simulink model "L400_sdofplant"  (R2024b)
settings: Solver=FixedStepAuto  StartTime=0  StopTime=200  FixedStep=5/1000  RelTol=1e-3
model workspace (MAT data in the model file):
  Sig : Simulink.Signal (value not decoded)
  Sig1 : Simulink.Signal (value not decoded)
  Sig2 : Simulink.Signal (value not decoded)
  Sig3 : Simulink.Signal (value not decoded)
  Sig4 : Simulink.Signal (value not decoded)
  Sig5 : Simulink.Signal (value not decoded)
  Sig6 : Simulink.Signal (value not decoded)
undefined symbols (not defined in the file or in its folder): convertTo, datetime, db, Earth, F, Light, MIL, motor, WGS84, WMM2020
libraries: aerolibconvert2 x6, aerolibasang x5, aerolibwind2 x3, aerolibactuator x2, aerolibtransform2 x2, shared6dof x1, matrix_library x1, aerolibatmos2 x1, aerolibgravity2 x1
(part 2 of 3)

== system L400_sdofplant/actuator/aerodynamic/actuator ==
  BusElementIn1 : Inport  PortName=command  Element=DAL
  BusElementIn : Inport  PortName=command  Element=DAL
  BusElementIn2 : Inport  PortName=command  Element=DER
  BusElementIn3 : Inport  PortName=command  Element=DR
  BusElementIn4 : Inport  PortName=command  Element=DEM
  BusElementIn5 : Inport  PortName=command  Element=DEL
  BusElementIn6 : Inport  PortName=command  Element=DFLO
  BusElementIn7 : Inport  PortName=command  Element=DFLI
  BusElementIn8 : Inport  PortName=command  Element=DFRI
  BusElementIn9 : Inport  PortName=command  Element=DFRO
  Data Type Conversion : DataTypeConversion  SaturateOnIntegerOverflow=off  RndMeth=Floor
  Demux : Demux  Outputs=10
  Mux : Mux  Inputs=10
  Saturation : Saturate  UpperLimit=[30,30,30,30,15,15,17,17,17,23]  LowerLimit=[0,0,0,0,-23,-23,-23,-23,-23,-23]
  Signal Specification4 : SignalSpecification  Unit=deg
  Variant Subsystem : Subsystem  Variant=on
  Bus Element Out : Outport  PortName=surface  Element=DFLO
  Bus Element Out1 : Outport  PortName=surface  Element=DFLI
  Bus Element Out2 : Outport  PortName=surface  Element=DFRI
  Bus Element Out3 : Outport  PortName=surface  Element=DFRO
  Bus Element Out4 : Outport  PortName=surface  Element=DAL
  Bus Element Out5 : Outport  PortName=surface  Element=DAR
  Bus Element Out6 : Outport  PortName=surface  Element=DEL
  Bus Element Out7 : Outport  PortName=surface  Element=DEM
  Bus Element Out8 : Outport  PortName=surface  Element=DER
  Bus Element Out9 : Outport  PortName=surface  Element=DR
  wires:
  Mux/1 -> Data Type Conversion/1
  Saturation/1 -> Signal Specification4/1
  Variant Subsystem/1(Out1) -> Demux/1
  Demux/1 -> Bus Element Out/1
  Demux/2 -> Bus Element Out1/1
  Demux/4 -> Bus Element Out3/1
  Demux/3 -> Bus Element Out2/1
  Signal Specification4/1 -> Variant Subsystem/1(In1)
  BusElementIn6/1 -> Mux/1
  BusElementIn7/1 -> Mux/2
  BusElementIn8/1 -> Mux/3
  BusElementIn9/1 -> Mux/4
  BusElementIn3/1 -> Mux/10
  BusElementIn2/1 -> Mux/9
  BusElementIn5/1 -> Mux/7
  BusElementIn4/1 -> Mux/8
  BusElementIn/1 -> Mux/6
  BusElementIn1/1 -> Mux/5
  Demux/5 -> Bus Element Out4/1
  Demux/6 -> Bus Element Out5/1
  Demux/7 -> Bus Element Out6/1
  Demux/8 -> Bus Element Out7/1
  Demux/9 -> Bus Element Out8/1
  Demux/10 -> Bus Element Out9/1
  Data Type Conversion/1 -> Saturation/1

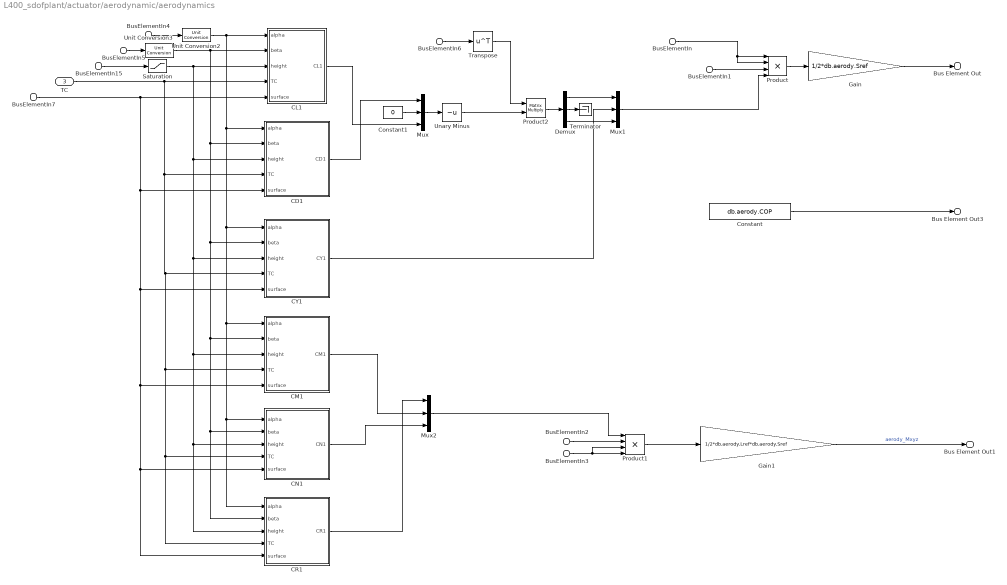
== system L400_sdofplant/actuator/aerodynamic/aerodynamics ==
  BusElementIn7 : Inport  PortName=surface
  BusElementIn : Inport  Port=2  PortName=state  Element=aircraft.airdata.airspeed
  BusElementIn3 : Inport  Port=2  PortName=state  Element=aircraft.airdata.airspeed
  BusElementIn4 : Inport  Port=2  PortName=state  Element=aircraft.airdata.alpha
  BusElementIn5 : Inport  Port=2  PortName=state  Element=aircraft.airdata.beta
  BusElementIn6 : Inport  Port=2  PortName=state  Element=aircraft.airdata.Rwb
  BusElementIn15 : Inport  Port=2  PortName=state  Element=aircraft.position.agl
  BusElementIn1 : Inport  Port=2  PortName=state  Element=environ.atmosphere.density
  BusElementIn2 : Inport  Port=2  PortName=state  Element=environ.atmosphere.density
  TC : Inport  Port=3
  CD1 : Subsystem
  CL1 : Subsystem
  CM1 : Subsystem
  CN1 : Subsystem
  CR1 : Subsystem
  CY1 : Subsystem
  Constant : Constant  Value=db.aerody.COP
  Constant1 : Constant  Value=0
  Demux : Demux  Outputs=3
  Gain : Gain  Gain=1/2*db.aerody.Sref
  Gain1 : Gain  Gain=1/2*db.aerody.Lref*db.aerody.Sref
  Mux : Mux  Inputs=3
  Mux1 : Mux  Inputs=3
  Mux2 : Mux  Inputs=3
  Product : Product  Inputs=4
  Product1 : Product  Inputs=4
  Product2 : Product  Multiplication=Matrix(*)
  Saturation : Saturate  UpperLimit=5.8  LowerLimit=0
  Terminator : Terminator
  Transpose : Math  Operator=transpose
  Unary Minus : UnaryMinus
  Unit Conversion2 : UnitConversion
  Unit Conversion3 : UnitConversion
  Bus Element Out : Outport  PortName=aerody  Element=Fxyz
  Bus Element Out1 : Outport  PortName=aerody  Element=Mxyz
  Bus Element Out3 : Outport  PortName=aerody  Element=Pxyz
  wires:
  BusElementIn/1 -> Product/2, Product/1
  BusElementIn2/1 -> Product1/2
  Constant/1 -> Bus Element Out3/1
  Product1/1 -> Gain1/1
  Product/1 -> Gain/1
  BusElementIn3/1 -> Product1/4, Product1/3
  Mux2/1 -> Product1/1
  BusElementIn1/1 -> Product/3
  Gain1/1 -> Bus Element Out1/1  "aerody_Mxyz"
  Unit Conversion2/1 -> CR1/1(alpha), CN1/1(alpha), CM1/1(alpha), CY1/1(alpha), CD1/1(alpha), CL1/1(alpha)
  BusElementIn7/1 -> CL1/5(surface), CD1/5(surface), CM1/5(surface), CN1/5(surface), CR1/5(surface), CY1/5(surface)
  BusElementIn4/1 -> Unit Conversion2/1
  BusElementIn5/1 -> Unit Conversion3/1
  BusElementIn15/1 -> Saturation/1
  TC/1 -> CM1/4(TC), CN1/4(TC), CR1/4(TC), CY1/4(TC), CD1/4(TC), CL1/4(TC)
  Unit Conversion3/1 -> CM1/2(beta), CN1/2(beta), CR1/2(beta), CY1/2(beta), CD1/2(beta), CL1/2(beta)
  CD1/1(CD1) -> Mux/1
  CL1/1(CL1) -> Mux/3
  Constant1/1 -> Mux/2
  Mux/1 -> Unary Minus/1
  BusElementIn6/1 -> Transpose/1
  Transpose/1 -> Product2/1
  CY1/1(CY1) -> Mux1/2
  Product2/1 -> Demux/1
  Demux/1 -> Mux1/1
  Demux/3 -> Mux1/3
  Demux/2 -> Terminator/1
  Mux1/1 -> Product/4
  CM1/1(CM1) -> Mux2/2
  CR1/1(CR1) -> Mux2/1
  CN1/1(CN1) -> Mux2/3
  Saturation/1 -> CM1/3(height), CN1/3(height), CR1/3(height), CY1/3(height), CD1/3(height), CL1/3(height)
  Unary Minus/1 -> Product2/2
  Gain/1 -> Bus Element Out/1

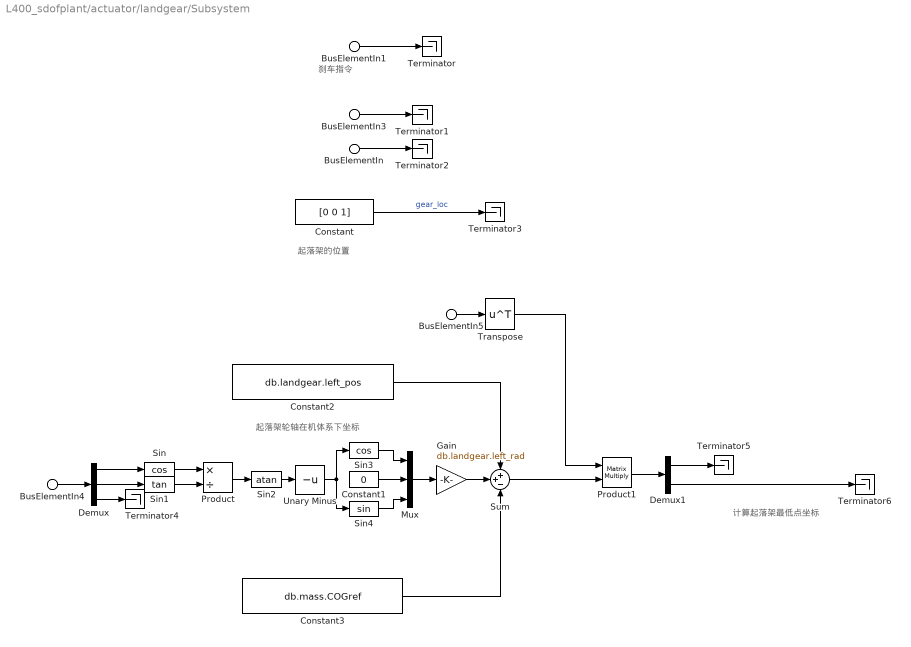
== system L400_sdofplant/actuator/landgear/Subsystem ==
  note: 起落架轮轴在机体系下坐标
  note: 计算起落架最低点坐标
  note: 刹车指令
  note: 起落架的位置
  BusElementIn1 : Inport  PortName=cmd  Element=DB
  BusElementIn : Inport  Port=2  PortName=state  Element=aircraft.position.agl
  BusElementIn3 : Inport  Port=2  PortName=state  Element=aircraft.position.alt
  BusElementIn4 : Inport  Port=2  PortName=state  Element=aircraft.attitude.phi_theta_psi
  BusElementIn5 : Inport  Port=2  PortName=state  Element=aircraft.attitude.Rbe
  Constant : Constant  Value=[0 0 1]
  Constant1 : Constant  Value=0
  Constant2 : Constant  Value=db.landgear.left_pos
  Constant3 : Constant  Value=db.mass.COGref
  Demux : Demux  Outputs=3
  Demux1 : Demux  Outputs=[2, 1]
  Gain : Gain  Gain=db.landgear.left_rad
  Mux : Mux  Inputs=3
  Product : Product  Inputs=*/
  Product1 : Product  Multiplication=Matrix(*)
  Sin : Trigonometry  Operator=cos
  Sin1 : Trigonometry  Operator=tan
  Sin2 : Trigonometry  Operator=atan
  Sin3 : Trigonometry  Operator=cos
  Sin4 : Trigonometry
  Sum : Sum  Inputs=++-
  Terminator{,1..6} (7 alike) : Terminator
  Transpose : Math  Operator=transpose
  Unary Minus : UnaryMinus
  wires:
  Constant/1 -> Terminator3/1  "gear_loc"
  BusElementIn1/1 -> Terminator/1
  BusElementIn3/1 -> Terminator1/1
  BusElementIn/1 -> Terminator2/1
  BusElementIn4/1 -> Demux/1
  Demux/2 -> Sin1/1
  Demux/1 -> Sin/1
  Sin/1 -> Product/1
  Sin1/1 -> Product/2
  Product/1 -> Sin2/1
  Demux/3 -> Terminator4/1
  Sin2/1 -> Unary Minus/1
  Constant1/1 -> Mux/2
  Sin3/1 -> Mux/1
  Sin4/1 -> Mux/3
  Mux/1 -> Gain/1
  BusElementIn5/1 -> Transpose/1
  Transpose/1 -> Product1/1
  Sum/1 -> Product1/2
  Unary Minus/1 -> Sin4/1, Sin3/1
  Constant2/1 -> Sum/1
  Gain/1 -> Sum/2
  Constant3/1 -> Sum/3
  Product1/1 -> Demux1/1
  Demux1/1 -> Terminator5/1
  Demux1/2 -> Terminator6/1

== system L400_sdofplant/force/Subsystem1/For Each Subsystem ==
  Fxyz : Inport  Partition=on  PartitionDimension=2  PartitionWidth=1  PartitionOffset=0
  Mxyz : Inport  Port=2  Partition=on  PartitionDimension=2  PartitionWidth=1  PartitionOffset=0
  Pxyz : Inport  Port=3  Partition=on  PartitionDimension=2  PartitionWidth=1  PartitionOffset=0
  COG : Inport  Port=4
  Cross Product : matrix_library/Cross Product
  For Each : ForEach  DisableCoverage=on
  Sum : Sum  Inputs=|+-
  Sum1 : Sum  Inputs=|++
  M : Outport  ConcatenationDimension=2
  wires:
  Mxyz/1 -> Sum1/2
  Sum/1 -> Cross Product/1
  Fxyz/1 -> Cross Product/2
  Sum1/1 -> M/1
  Cross Product/1 -> Sum1/1
  Pxyz/1 -> Sum/1
  COG/1 -> Sum/2

== system L400_sdofplant/sensor/gps/posix time ==
  Clock : Clock
  Constant : Constant  Value=convertTo(datetime('now','TimeZone','UTC'),'posixtime')
  Gain : Gain  Gain=1e6  OutDataTypeStr=uint64
  Sum : Sum  Inputs=|++
  utc : Outport  Unit=µs
  wires:
  Clock/1 -> Sum/1
  Sum/1 -> Gain/1
  Constant/1 -> Sum/2
  Gain/1 -> utc/1

== system L400_sdofplant/state/Variant Subsystem/Subsystem ==
  h(m) : Inport
  μ(deg) : Inport  Port=2
  l(deg) : Inport  Port=3
  Constant : Constant  Value=[1 0 0]
  Constant1 : Constant  Value=0
  Terminator : Terminator
  Terminator1 : Terminator
  Terminator2 : Terminator
  XYZ(nT) : Outport
  H(nT) : Outport  Port=2
  D(deg) : Outport  Port=3
  I(deg) : Outport  Port=4
  F(nT) : Outport  Port=5
  wires:
  h(m)/1 -> Terminator/1
  l(deg)/1 -> Terminator2/1
  μ(deg)/1 -> Terminator1/1
  Constant/1 -> XYZ(nT)/1
  Constant1/1 -> F(nT)/1, I(deg)/1, H(nT)/1, D(deg)/1

== system L400_sdofplant/state/Variant Subsystem/Subsystem1 ==
  h(m) : Inport
  μ(deg) : Inport  Port=2
  l(deg) : Inport  Port=3
  World Magnetic Model : aerolibgravity2/World Magnetic Model  model=WMM2020 (2020-2025)  customFile='WMM2020.COF'  units=Metric (MKS)  time_in=off  month=January  day=1  year=2020  action=Error  h_out=on  dec_out=on  inc_out=on  ti_out=on
  XYZ(nT) : Outport
  H(nT) : Outport  Port=2
  D(deg) : Outport  Port=3
  I(deg) : Outport  Port=4
  F(nT) : Outport  Port=5
  wires:
  h(m)/1 -> World Magnetic Model/1
  World Magnetic Model/1 -> XYZ(nT)/1
  World Magnetic Model/2 -> H(nT)/1
  World Magnetic Model/3 -> D(deg)/1
  World Magnetic Model/4 -> I(deg)/1
  World Magnetic Model/5 -> F(nT)/1
  l(deg)/1 -> World Magnetic Model/3
  μ(deg)/1 -> World Magnetic Model/2

== system L400_sdofplant/actuator/aerodynamic/actuator/Variant Subsystem ==
  note: 1) Add Subsystem or Model blocks as valid variant choices.
      | 2) You cannot connect blocks at this level. At simulation, connectivity is automatically
      | determined, based on the active variant and port name matching.
  In1 : Inport
  Subsystem : Subsystem  VariantControl=true
  Subsystem1 : Subsystem  VariantControl=false
  Out1 : Outport

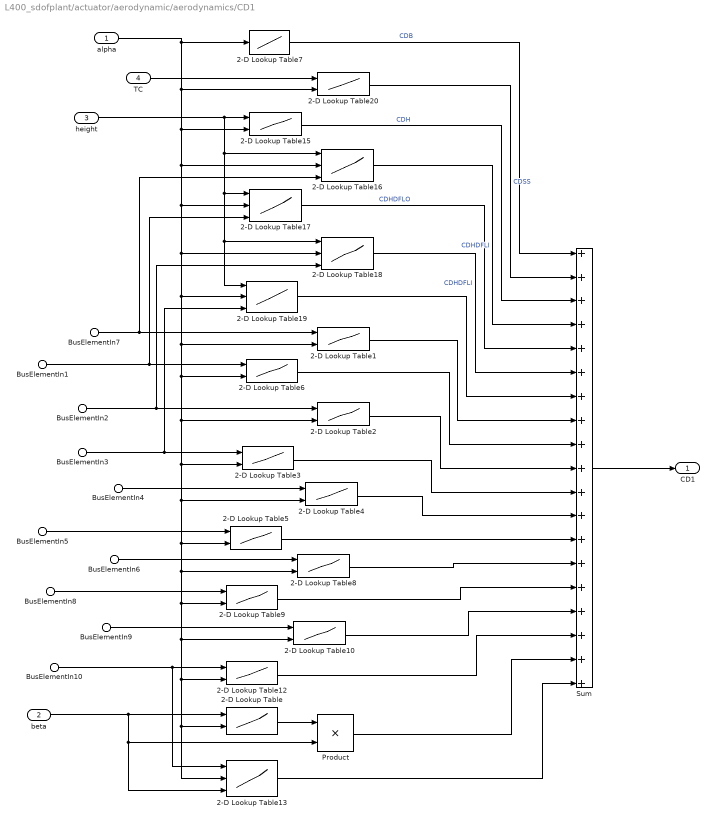
== system L400_sdofplant/actuator/aerodynamic/aerodynamics/CD1 ==
  alpha : Inport  Unit=deg
  beta : Inport  Port=2  Unit=deg
  height : Inport  Port=3
  TC : Inport  Port=4
  BusElementIn7 : Inport  Port=5  PortName=surface  Element=DFLI
  BusElementIn1 : Inport  Port=5  PortName=surface  Element=DFLO
  BusElementIn2 : Inport  Port=5  PortName=surface  Element=DFRI
  BusElementIn3 : Inport  Port=5  PortName=surface  Element=DFRO
  BusElementIn4 : Inport  Port=5  PortName=surface  Element=DAL
  BusElementIn5 : Inport  Port=5  PortName=surface  Element=DAR
  BusElementIn6 : Inport  Port=5  PortName=surface  Element=DEL
  BusElementIn8 : Inport  Port=5  PortName=surface  Element=DEM
  BusElementIn9 : Inport  Port=5  PortName=surface  Element=DER
  BusElementIn10 : Inport  Port=5  PortName=surface  Element=DR
  2-D Lookup Table : Lookup_n-D  LookupTableObject=''  BreakpointsForDimension1=db.aerody.VBETA  BreakpointsForDimension2=db.aerody.VALPHA  BreakpointsForDimension1FirstPoint=10  BreakpointsForDimension2FirstPoint=10  BreakpointsForDimension1Spacing=12  BreakpointsForDimension2Spacing=12  IndexSearchMethod=Linear search  BeginIndexSearchUsingPreviousIndexResult=on  Table=db.aerody.DCDBETA  ExtrapMethod=Clip  DiagnosticForOutOfRangeInput=Warning  InternalRulePriority=Speed  RndMeth=Simplest
      settings: InputPortMap=u0,u1
  2-D Lookup Table1 : Lookup_n-D  LookupTableObject=''  BreakpointsForDimension1=db.aerody.VDF  BreakpointsForDimension2=db.aerody.VALPHA  BreakpointsForDimension1FirstPoint=10  BreakpointsForDimension2FirstPoint=10  BreakpointsForDimension1Spacing=12  BreakpointsForDimension2Spacing=12  IndexSearchMethod=Linear search  BeginIndexSearchUsingPreviousIndexResult=on  Table=db.aerody.CDDFLI  ExtrapMethod=Clip  DiagnosticForOutOfRangeInput=Warning  InternalRulePriority=Speed  RndMeth=Simplest
      settings: InputPortMap=u0,u1
  2-D Lookup Table10 : Lookup_n-D  LookupTableObject=''  BreakpointsForDimension1=db.aerody.VDE  BreakpointsForDimension2=db.aerody.VALPHA  BreakpointsForDimension1FirstPoint=10  BreakpointsForDimension2FirstPoint=10  BreakpointsForDimension1Spacing=12  BreakpointsForDimension2Spacing=12  IndexSearchMethod=Linear search  BeginIndexSearchUsingPreviousIndexResult=on  Table=db.aerody.CDDER  ExtrapMethod=Clip  DiagnosticForOutOfRangeInput=Warning  InternalRulePriority=Speed  RndMeth=Simplest
      settings: InputPortMap=u0,u1
  2-D Lookup Table12 : Lookup_n-D  LookupTableObject=''  BreakpointsForDimension1=db.aerody.VDR  BreakpointsForDimension2=db.aerody.VALPHA  BreakpointsForDimension1FirstPoint=10  BreakpointsForDimension2FirstPoint=10  BreakpointsForDimension1Spacing=12  BreakpointsForDimension2Spacing=12  IndexSearchMethod=Linear search  BeginIndexSearchUsingPreviousIndexResult=on  Table=db.aerody.CDDR  ExtrapMethod=Clip  DiagnosticForOutOfRangeInput=Warning  InternalRulePriority=Speed  RndMeth=Simplest
      settings: InputPortMap=u0,u1
  2-D Lookup Table13 : Lookup_n-D  NumberOfTableDimensions=3  LookupTableObject=''  BreakpointsForDimension1=db.aerody.VDR  BreakpointsForDimension2=db.aerody.VALPHA  BreakpointsForDimension3=db.aerody.VBETA  BreakpointsForDimension1FirstPoint=10  BreakpointsForDimension2FirstPoint=10  BreakpointsForDimension1Spacing=12  BreakpointsForDimension2Spacing=12  IndexSearchMethod=Linear search  BeginIndexSearchUsingPreviousIndexResult=on  Table=db.aerody.CDDRBETA  ExtrapMethod=Clip  DiagnosticForOutOfRangeInput=Warning  InternalRulePriority=Speed  RndMeth=Simplest
      settings: InputPortMap=u0,u1,u2
  2-D Lookup Table15 : Lookup_n-D  LookupTableObject=''  BreakpointsForDimension1=db.aerody.VH  BreakpointsForDimension2=db.aerody.VALPHA  BreakpointsForDimension1FirstPoint=10  BreakpointsForDimension2FirstPoint=10  BreakpointsForDimension1Spacing=12  BreakpointsForDimension2Spacing=12  IndexSearchMethod=Linear search  BeginIndexSearchUsingPreviousIndexResult=on  Table=db.aerody.CDH  ExtrapMethod=Clip  DiagnosticForOutOfRangeInput=Warning  InternalRulePriority=Speed  RndMeth=Simplest
      settings: InputPortMap=u0,u1
  2-D Lookup Table16 : Lookup_n-D  NumberOfTableDimensions=3  LookupTableObject=''  BreakpointsForDimension1=db.aerody.VH  BreakpointsForDimension2=db.aerody.VALPHA  BreakpointsForDimension3=db.aerody.VDF  BreakpointsForDimension1FirstPoint=10  BreakpointsForDimension2FirstPoint=10  BreakpointsForDimension1Spacing=12  BreakpointsForDimension2Spacing=12  IndexSearchMethod=Linear search  BeginIndexSearchUsingPreviousIndexResult=on  Table=db.aerody.CDHDFLI  ExtrapMethod=Clip  DiagnosticForOutOfRangeInput=Warning  InternalRulePriority=Speed  RndMeth=Simplest
      settings: InputPortMap=u0,u1,u2
  2-D Lookup Table17 : Lookup_n-D  NumberOfTableDimensions=3  LookupTableObject=''  BreakpointsForDimension1=db.aerody.VH  BreakpointsForDimension2=db.aerody.VALPHA  BreakpointsForDimension3=db.aerody.VDF  BreakpointsForDimension1FirstPoint=10  BreakpointsForDimension2FirstPoint=10  BreakpointsForDimension1Spacing=12  BreakpointsForDimension2Spacing=12  IndexSearchMethod=Linear search  BeginIndexSearchUsingPreviousIndexResult=on  Table=db.aerody.CDHDFLO  ExtrapMethod=Clip  DiagnosticForOutOfRangeInput=Warning  InternalRulePriority=Speed  RndMeth=Simplest
      settings: InputPortMap=u0,u1,u2
  2-D Lookup Table18 : Lookup_n-D  NumberOfTableDimensions=3  LookupTableObject=''  BreakpointsForDimension1=db.aerody.VH  BreakpointsForDimension2=db.aerody.VALPHA  BreakpointsForDimension3=db.aerody.VDF  BreakpointsForDimension1FirstPoint=10  BreakpointsForDimension2FirstPoint=10  BreakpointsForDimension1Spacing=12  BreakpointsForDimension2Spacing=12  IndexSearchMethod=Linear search  BeginIndexSearchUsingPreviousIndexResult=on  Table=db.aerody.CDHDFRI  ExtrapMethod=Clip  DiagnosticForOutOfRangeInput=Warning  InternalRulePriority=Speed  RndMeth=Simplest
      settings: InputPortMap=u0,u1,u2
  2-D Lookup Table19 : Lookup_n-D  NumberOfTableDimensions=3  LookupTableObject=''  BreakpointsForDimension1=db.aerody.VH  BreakpointsForDimension2=db.aerody.VALPHA  BreakpointsForDimension3=db.aerody.VDF  BreakpointsForDimension1FirstPoint=10  BreakpointsForDimension2FirstPoint=10  BreakpointsForDimension1Spacing=12  BreakpointsForDimension2Spacing=12  IndexSearchMethod=Linear search  BeginIndexSearchUsingPreviousIndexResult=on  Table=db.aerody.CDHDFRO  ExtrapMethod=Clip  DiagnosticForOutOfRangeInput=Warning  InternalRulePriority=Speed  RndMeth=Simplest
      settings: InputPortMap=u0,u1,u2
  2-D Lookup Table2 : Lookup_n-D  LookupTableObject=''  BreakpointsForDimension1=db.aerody.VDF  BreakpointsForDimension2=db.aerody.VALPHA  BreakpointsForDimension1FirstPoint=10  BreakpointsForDimension2FirstPoint=10  BreakpointsForDimension1Spacing=12  BreakpointsForDimension2Spacing=12  IndexSearchMethod=Linear search  BeginIndexSearchUsingPreviousIndexResult=on  Table=db.aerody.CDDFRI  ExtrapMethod=Clip  DiagnosticForOutOfRangeInput=Warning  InternalRulePriority=Speed  RndMeth=Simplest
      settings: InputPortMap=u0,u1
  2-D Lookup Table20 : Lookup_n-D  LookupTableObject=''  BreakpointsForDimension1=db.aerody.VTC  BreakpointsForDimension2=db.aerody.VALPHA  BreakpointsForDimension1FirstPoint=10  BreakpointsForDimension2FirstPoint=10  BreakpointsForDimension1Spacing=12  BreakpointsForDimension2Spacing=12  IndexSearchMethod=Linear search  BeginIndexSearchUsingPreviousIndexResult=on  Table=db.aerody.CDSS  ExtrapMethod=Clip  DiagnosticForOutOfRangeInput=Warning  InternalRulePriority=Speed  RndMeth=Simplest
      settings: InputPortMap=u0,u1
  2-D Lookup Table3 : Lookup_n-D  LookupTableObject=''  BreakpointsForDimension1=db.aerody.VDF  BreakpointsForDimension2=db.aerody.VALPHA  BreakpointsForDimension1FirstPoint=10  BreakpointsForDimension2FirstPoint=10  BreakpointsForDimension1Spacing=12  BreakpointsForDimension2Spacing=12  IndexSearchMethod=Linear search  BeginIndexSearchUsingPreviousIndexResult=on  Table=db.aerody.CDDFRO  ExtrapMethod=Clip  DiagnosticForOutOfRangeInput=Warning  InternalRulePriority=Speed  RndMeth=Simplest
      settings: InputPortMap=u0,u1
  2-D Lookup Table4 : Lookup_n-D  LookupTableObject=''  BreakpointsForDimension1=db.aerody.VDA  BreakpointsForDimension2=db.aerody.VALPHA  BreakpointsForDimension1FirstPoint=10  BreakpointsForDimension2FirstPoint=10  BreakpointsForDimension1Spacing=12  BreakpointsForDimension2Spacing=12  IndexSearchMethod=Linear search  BeginIndexSearchUsingPreviousIndexResult=on  Table=db.aerody.CDDAL  ExtrapMethod=Clip  DiagnosticForOutOfRangeInput=Warning  InternalRulePriority=Speed  RndMeth=Simplest
      settings: InputPortMap=u0,u1
  2-D Lookup Table5 : Lookup_n-D  LookupTableObject=''  BreakpointsForDimension1=db.aerody.VDA  BreakpointsForDimension2=db.aerody.VALPHA  BreakpointsForDimension1FirstPoint=10  BreakpointsForDimension2FirstPoint=10  BreakpointsForDimension1Spacing=12  BreakpointsForDimension2Spacing=12  IndexSearchMethod=Linear search  BeginIndexSearchUsingPreviousIndexResult=on  Table=db.aerody.CDDAR  ExtrapMethod=Clip  DiagnosticForOutOfRangeInput=Warning  InternalRulePriority=Speed  RndMeth=Simplest
      settings: InputPortMap=u0,u1
  2-D Lookup Table6 : Lookup_n-D  LookupTableObject=''  BreakpointsForDimension1=db.aerody.VDF  BreakpointsForDimension2=db.aerody.VALPHA  BreakpointsForDimension1FirstPoint=10  BreakpointsForDimension2FirstPoint=10  BreakpointsForDimension1Spacing=12  BreakpointsForDimension2Spacing=12  IndexSearchMethod=Linear search  BeginIndexSearchUsingPreviousIndexResult=on  Table=db.aerody.CDDFLO  ExtrapMethod=Clip  DiagnosticForOutOfRangeInput=Warning  InternalRulePriority=Speed  RndMeth=Simplest
      settings: InputPortMap=u0,u1
  2-D Lookup Table7 : Lookup_n-D  NumberOfTableDimensions=1  LookupTableObject=''  BreakpointsForDimension1=db.aerody.VALPHA  BreakpointsForDimension2=aerody.basic.cx.beta  BreakpointsForDimension1FirstPoint=10  BreakpointsForDimension2FirstPoint=10  BreakpointsForDimension1Spacing=12  BreakpointsForDimension2Spacing=12  IndexSearchMethod=Linear search  BeginIndexSearchUsingPreviousIndexResult=on  Table=db.aerody.CDB  ExtrapMethod=Clip  DiagnosticForOutOfRangeInput=Warning  InternalRulePriority=Speed  RndMeth=Simplest
  2-D Lookup Table8 : Lookup_n-D  LookupTableObject=''  BreakpointsForDimension1=db.aerody.VDE  BreakpointsForDimension2=db.aerody.VALPHA  BreakpointsForDimension1FirstPoint=10  BreakpointsForDimension2FirstPoint=10  BreakpointsForDimension1Spacing=12  BreakpointsForDimension2Spacing=12  IndexSearchMethod=Linear search  BeginIndexSearchUsingPreviousIndexResult=on  Table=db.aerody.CDDEL  ExtrapMethod=Clip  DiagnosticForOutOfRangeInput=Warning  InternalRulePriority=Speed  RndMeth=Simplest
      settings: InputPortMap=u0,u1
  2-D Lookup Table9 : Lookup_n-D  LookupTableObject=''  BreakpointsForDimension1=db.aerody.VDE  BreakpointsForDimension2=db.aerody.VALPHA  BreakpointsForDimension1FirstPoint=10  BreakpointsForDimension2FirstPoint=10  BreakpointsForDimension1Spacing=12  BreakpointsForDimension2Spacing=12  IndexSearchMethod=Linear search  BeginIndexSearchUsingPreviousIndexResult=on  Table=db.aerody.CDDEM  ExtrapMethod=Clip  DiagnosticForOutOfRangeInput=Warning  InternalRulePriority=Speed  RndMeth=Simplest
      settings: InputPortMap=u0,u1
  Product : Product
  Sum : Sum  Inputs=19
  CD1 : Outport
  wires:
  alpha/1 -> 2-D Lookup Table7/1, 2-D Lookup Table20/2, 2-D Lookup Table15/2, 2-D Lookup Table16/2, 2-D Lookup Table17/2, 2-D Lookup Table18/2, 2-D Lookup Table19/2, 2-D Lookup Table1/2, 2-D Lookup Table6/2, 2-D Lookup Table2/2, 2-D Lookup Table/2, 2-D Lookup Table13/2, 2-D Lookup Table12/2, 2-D Lookup Table10/2, 2-D Lookup Table9/2, 2-D Lookup Table8/2, 2-D Lookup Table5/2, 2-D Lookup Table4/2, 2-D Lookup Table3/2
  TC/1 -> 2-D Lookup Table20/1
  height/1 -> 2-D Lookup Table15/1, 2-D Lookup Table16/1, 2-D Lookup Table17/1, 2-D Lookup Table18/1, 2-D Lookup Table19/1
  2-D Lookup Table/1 -> Product/1
  beta/1 -> 2-D Lookup Table13/3, Product/2, 2-D Lookup Table/1
  BusElementIn10/1 -> 2-D Lookup Table13/1, 2-D Lookup Table12/1
  BusElementIn9/1 -> 2-D Lookup Table10/1
  BusElementIn8/1 -> 2-D Lookup Table9/1
  BusElementIn6/1 -> 2-D Lookup Table8/1
  BusElementIn5/1 -> 2-D Lookup Table5/1
  BusElementIn4/1 -> 2-D Lookup Table4/1
  BusElementIn3/1 -> 2-D Lookup Table19/3, 2-D Lookup Table3/1
  BusElementIn2/1 -> 2-D Lookup Table18/3, 2-D Lookup Table2/1
  BusElementIn1/1 -> 2-D Lookup Table17/3, 2-D Lookup Table6/1
  BusElementIn7/1 -> 2-D Lookup Table16/3, 2-D Lookup Table1/1
  Sum/1 -> CD1/1
  2-D Lookup Table4/1 -> Sum/12
  2-D Lookup Table8/1 -> Sum/14
  2-D Lookup Table2/1 -> Sum/10
  2-D Lookup Table1/1 -> Sum/8
  2-D Lookup Table10/1 -> Sum/16
  2-D Lookup Table5/1 -> Sum/13
  2-D Lookup Table3/1 -> Sum/11
  2-D Lookup Table18/1 -> Sum/6  "CDHDFLI"
  2-D Lookup Table9/1 -> Sum/15
  2-D Lookup Table6/1 -> Sum/9
  2-D Lookup Table16/1 -> Sum/4  "CDHDFLI"
  Product/1 -> Sum/18
  2-D Lookup Table12/1 -> Sum/17
  2-D Lookup Table19/1 -> Sum/7
  2-D Lookup Table20/1 -> Sum/2  "CDSS"
  2-D Lookup Table17/1 -> Sum/5  "CDHDFLO"
  2-D Lookup Table15/1 -> Sum/3  "CDH"
  2-D Lookup Table13/1 -> Sum/19
  2-D Lookup Table7/1 -> Sum/1  "CDB"

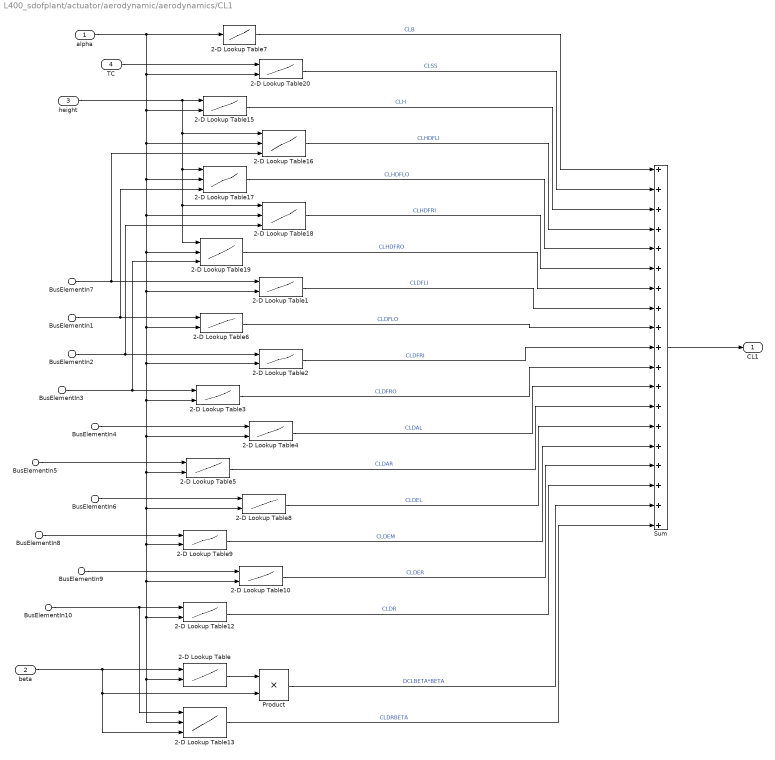
== system L400_sdofplant/actuator/aerodynamic/aerodynamics/CL1 ==
  alpha : Inport  Unit=deg
  beta : Inport  Port=2  Unit=deg
  height : Inport  Port=3
  TC : Inport  Port=4
  BusElementIn7 : Inport  Port=5  PortName=surface  Element=DFLI
  BusElementIn1 : Inport  Port=5  PortName=surface  Element=DFLO
  BusElementIn2 : Inport  Port=5  PortName=surface  Element=DFRI
  BusElementIn3 : Inport  Port=5  PortName=surface  Element=DFRO
  BusElementIn4 : Inport  Port=5  PortName=surface  Element=DAL
  BusElementIn5 : Inport  Port=5  PortName=surface  Element=DAR
  BusElementIn6 : Inport  Port=5  PortName=surface  Element=DEL
  BusElementIn8 : Inport  Port=5  PortName=surface  Element=DEM
  BusElementIn9 : Inport  Port=5  PortName=surface  Element=DER
  BusElementIn10 : Inport  Port=5  PortName=surface  Element=DR
  2-D Lookup Table : Lookup_n-D  LookupTableObject=''  BreakpointsForDimension1=db.aerody.VBETA  BreakpointsForDimension2=db.aerody.VALPHA  BreakpointsForDimension1FirstPoint=10  BreakpointsForDimension2FirstPoint=10  BreakpointsForDimension1Spacing=12  BreakpointsForDimension2Spacing=12  IndexSearchMethod=Linear search  BeginIndexSearchUsingPreviousIndexResult=on  Table=db.aerody.DCLBETA  ExtrapMethod=Clip  DiagnosticForOutOfRangeInput=Warning  InternalRulePriority=Speed  RndMeth=Simplest
      settings: InputPortMap=u0,u1
  2-D Lookup Table1 : Lookup_n-D  LookupTableObject=''  BreakpointsForDimension1=db.aerody.VDF  BreakpointsForDimension2=db.aerody.VALPHA  BreakpointsForDimension1FirstPoint=10  BreakpointsForDimension2FirstPoint=10  BreakpointsForDimension1Spacing=12  BreakpointsForDimension2Spacing=12  IndexSearchMethod=Linear search  BeginIndexSearchUsingPreviousIndexResult=on  Table=db.aerody.CLDFLI  ExtrapMethod=Clip  DiagnosticForOutOfRangeInput=Warning  InternalRulePriority=Speed  RndMeth=Simplest
      settings: InputPortMap=u0,u1
  2-D Lookup Table10 : Lookup_n-D  LookupTableObject=''  BreakpointsForDimension1=db.aerody.VDE  BreakpointsForDimension2=db.aerody.VALPHA  BreakpointsForDimension1FirstPoint=10  BreakpointsForDimension2FirstPoint=10  BreakpointsForDimension1Spacing=12  BreakpointsForDimension2Spacing=12  IndexSearchMethod=Linear search  BeginIndexSearchUsingPreviousIndexResult=on  Table=db.aerody.CLDER  ExtrapMethod=Clip  DiagnosticForOutOfRangeInput=Warning  InternalRulePriority=Speed  RndMeth=Simplest
      settings: InputPortMap=u0,u1
  2-D Lookup Table12 : Lookup_n-D  LookupTableObject=''  BreakpointsForDimension1=db.aerody.VDR  BreakpointsForDimension2=db.aerody.VALPHA  BreakpointsForDimension1FirstPoint=10  BreakpointsForDimension2FirstPoint=10  BreakpointsForDimension1Spacing=12  BreakpointsForDimension2Spacing=12  IndexSearchMethod=Linear search  BeginIndexSearchUsingPreviousIndexResult=on  Table=db.aerody.CLDR  ExtrapMethod=Clip  DiagnosticForOutOfRangeInput=Warning  InternalRulePriority=Speed  RndMeth=Simplest
      settings: InputPortMap=u0,u1
  2-D Lookup Table13 : Lookup_n-D  NumberOfTableDimensions=3  LookupTableObject=''  BreakpointsForDimension1=db.aerody.VDR  BreakpointsForDimension2=db.aerody.VALPHA  BreakpointsForDimension3=db.aerody.VBETA  BreakpointsForDimension1FirstPoint=10  BreakpointsForDimension2FirstPoint=10  BreakpointsForDimension1Spacing=12  BreakpointsForDimension2Spacing=12  IndexSearchMethod=Linear search  BeginIndexSearchUsingPreviousIndexResult=on  Table=db.aerody.CLDRBETA  ExtrapMethod=Clip  DiagnosticForOutOfRangeInput=Warning  InternalRulePriority=Speed  RndMeth=Simplest
      settings: InputPortMap=u0,u1,u2
  2-D Lookup Table15 : Lookup_n-D  LookupTableObject=''  BreakpointsForDimension1=db.aerody.VH  BreakpointsForDimension2=db.aerody.VALPHA  BreakpointsForDimension1FirstPoint=10  BreakpointsForDimension2FirstPoint=10  BreakpointsForDimension1Spacing=12  BreakpointsForDimension2Spacing=12  IndexSearchMethod=Linear search  BeginIndexSearchUsingPreviousIndexResult=on  Table=db.aerody.CLH  ExtrapMethod=Clip  DiagnosticForOutOfRangeInput=Warning  InternalRulePriority=Speed  RndMeth=Simplest
      settings: InputPortMap=u0,u1
  2-D Lookup Table16 : Lookup_n-D  NumberOfTableDimensions=3  LookupTableObject=''  BreakpointsForDimension1=db.aerody.VH  BreakpointsForDimension2=db.aerody.VALPHA  BreakpointsForDimension3=db.aerody.VDF  BreakpointsForDimension1FirstPoint=10  BreakpointsForDimension2FirstPoint=10  BreakpointsForDimension1Spacing=12  BreakpointsForDimension2Spacing=12  IndexSearchMethod=Linear search  BeginIndexSearchUsingPreviousIndexResult=on  Table=db.aerody.CLHDFLI  ExtrapMethod=Clip  DiagnosticForOutOfRangeInput=Warning  InternalRulePriority=Speed  RndMeth=Simplest
      settings: InputPortMap=u0,u1,u2
  2-D Lookup Table17 : Lookup_n-D  NumberOfTableDimensions=3  LookupTableObject=''  BreakpointsForDimension1=db.aerody.VH  BreakpointsForDimension2=db.aerody.VALPHA  BreakpointsForDimension3=db.aerody.VDF  BreakpointsForDimension1FirstPoint=10  BreakpointsForDimension2FirstPoint=10  BreakpointsForDimension1Spacing=12  BreakpointsForDimension2Spacing=12  IndexSearchMethod=Linear search  BeginIndexSearchUsingPreviousIndexResult=on  Table=db.aerody.CLHDFLO  ExtrapMethod=Clip  DiagnosticForOutOfRangeInput=Warning  InternalRulePriority=Speed  RndMeth=Simplest
      settings: InputPortMap=u0,u1,u2
  2-D Lookup Table18 : Lookup_n-D  NumberOfTableDimensions=3  LookupTableObject=''  BreakpointsForDimension1=db.aerody.VH  BreakpointsForDimension2=db.aerody.VALPHA  BreakpointsForDimension3=db.aerody.VDF  BreakpointsForDimension1FirstPoint=10  BreakpointsForDimension2FirstPoint=10  BreakpointsForDimension1Spacing=12  BreakpointsForDimension2Spacing=12  IndexSearchMethod=Linear search  BeginIndexSearchUsingPreviousIndexResult=on  Table=db.aerody.CLHDFRI  ExtrapMethod=Clip  DiagnosticForOutOfRangeInput=Warning  InternalRulePriority=Speed  RndMeth=Simplest
      settings: InputPortMap=u0,u1,u2
  2-D Lookup Table19 : Lookup_n-D  NumberOfTableDimensions=3  LookupTableObject=''  BreakpointsForDimension1=db.aerody.VH  BreakpointsForDimension2=db.aerody.VALPHA  BreakpointsForDimension3=db.aerody.VDF  BreakpointsForDimension1FirstPoint=10  BreakpointsForDimension2FirstPoint=10  BreakpointsForDimension1Spacing=12  BreakpointsForDimension2Spacing=12  IndexSearchMethod=Linear search  BeginIndexSearchUsingPreviousIndexResult=on  Table=db.aerody.CLHDFRO  ExtrapMethod=Clip  DiagnosticForOutOfRangeInput=Warning  InternalRulePriority=Speed  RndMeth=Simplest
      settings: InputPortMap=u0,u1,u2
  2-D Lookup Table2 : Lookup_n-D  LookupTableObject=''  BreakpointsForDimension1=db.aerody.VDF  BreakpointsForDimension2=db.aerody.VALPHA  BreakpointsForDimension1FirstPoint=10  BreakpointsForDimension2FirstPoint=10  BreakpointsForDimension1Spacing=12  BreakpointsForDimension2Spacing=12  IndexSearchMethod=Linear search  BeginIndexSearchUsingPreviousIndexResult=on  Table=db.aerody.CLDFRI  ExtrapMethod=Clip  DiagnosticForOutOfRangeInput=Warning  InternalRulePriority=Speed  RndMeth=Simplest
      settings: InputPortMap=u0,u1
  2-D Lookup Table20 : Lookup_n-D  LookupTableObject=''  BreakpointsForDimension1=db.aerody.VTC  BreakpointsForDimension2=db.aerody.VALPHA  BreakpointsForDimension1FirstPoint=10  BreakpointsForDimension2FirstPoint=10  BreakpointsForDimension1Spacing=12  BreakpointsForDimension2Spacing=12  IndexSearchMethod=Linear search  BeginIndexSearchUsingPreviousIndexResult=on  Table=db.aerody.CLSS  ExtrapMethod=Clip  DiagnosticForOutOfRangeInput=Warning  InternalRulePriority=Speed  RndMeth=Simplest
      settings: InputPortMap=u0,u1
  2-D Lookup Table3 : Lookup_n-D  LookupTableObject=''  BreakpointsForDimension1=db.aerody.VDF  BreakpointsForDimension2=db.aerody.VALPHA  BreakpointsForDimension1FirstPoint=10  BreakpointsForDimension2FirstPoint=10  BreakpointsForDimension1Spacing=12  BreakpointsForDimension2Spacing=12  IndexSearchMethod=Linear search  BeginIndexSearchUsingPreviousIndexResult=on  Table=db.aerody.CLDFRO  ExtrapMethod=Clip  DiagnosticForOutOfRangeInput=Warning  InternalRulePriority=Speed  RndMeth=Simplest
      settings: InputPortMap=u0,u1
  2-D Lookup Table4 : Lookup_n-D  LookupTableObject=''  BreakpointsForDimension1=db.aerody.VDA  BreakpointsForDimension2=db.aerody.VALPHA  BreakpointsForDimension1FirstPoint=10  BreakpointsForDimension2FirstPoint=10  BreakpointsForDimension1Spacing=12  BreakpointsForDimension2Spacing=12  IndexSearchMethod=Linear search  BeginIndexSearchUsingPreviousIndexResult=on  Table=db.aerody.CLDAL  ExtrapMethod=Clip  DiagnosticForOutOfRangeInput=Warning  InternalRulePriority=Speed  RndMeth=Simplest
      settings: InputPortMap=u0,u1
  2-D Lookup Table5 : Lookup_n-D  LookupTableObject=''  BreakpointsForDimension1=db.aerody.VDA  BreakpointsForDimension2=db.aerody.VALPHA  BreakpointsForDimension1FirstPoint=10  BreakpointsForDimension2FirstPoint=10  BreakpointsForDimension1Spacing=12  BreakpointsForDimension2Spacing=12  IndexSearchMethod=Linear search  BeginIndexSearchUsingPreviousIndexResult=on  Table=db.aerody.CLDAR  ExtrapMethod=Clip  DiagnosticForOutOfRangeInput=Warning  InternalRulePriority=Speed  RndMeth=Simplest
      settings: InputPortMap=u0,u1
  2-D Lookup Table6 : Lookup_n-D  LookupTableObject=''  BreakpointsForDimension1=db.aerody.VDF  BreakpointsForDimension2=db.aerody.VALPHA  BreakpointsForDimension1FirstPoint=10  BreakpointsForDimension2FirstPoint=10  BreakpointsForDimension1Spacing=12  BreakpointsForDimension2Spacing=12  IndexSearchMethod=Linear search  BeginIndexSearchUsingPreviousIndexResult=on  Table=db.aerody.CLDFLO  ExtrapMethod=Clip  DiagnosticForOutOfRangeInput=Warning  InternalRulePriority=Speed  RndMeth=Simplest
      settings: InputPortMap=u0,u1
  2-D Lookup Table7 : Lookup_n-D  NumberOfTableDimensions=1  LookupTableObject=''  BreakpointsForDimension1=db.aerody.VALPHA  BreakpointsForDimension2=aerody.basic.cx.beta  BreakpointsForDimension1FirstPoint=10  BreakpointsForDimension2FirstPoint=10  BreakpointsForDimension1Spacing=12  BreakpointsForDimension2Spacing=12  IndexSearchMethod=Linear search  BeginIndexSearchUsingPreviousIndexResult=on  Table=db.aerody.CLB  ExtrapMethod=Clip  DiagnosticForOutOfRangeInput=Warning  InternalRulePriority=Speed  RndMeth=Simplest
  2-D Lookup Table8 : Lookup_n-D  LookupTableObject=''  BreakpointsForDimension1=db.aerody.VDE  BreakpointsForDimension2=db.aerody.VALPHA  BreakpointsForDimension1FirstPoint=10  BreakpointsForDimension2FirstPoint=10  BreakpointsForDimension1Spacing=12  BreakpointsForDimension2Spacing=12  IndexSearchMethod=Linear search  BeginIndexSearchUsingPreviousIndexResult=on  Table=db.aerody.CLDEL  ExtrapMethod=Clip  DiagnosticForOutOfRangeInput=Warning  InternalRulePriority=Speed  RndMeth=Simplest
      settings: InputPortMap=u0,u1
  2-D Lookup Table9 : Lookup_n-D  LookupTableObject=''  BreakpointsForDimension1=db.aerody.VDE  BreakpointsForDimension2=db.aerody.VALPHA  BreakpointsForDimension1FirstPoint=10  BreakpointsForDimension2FirstPoint=10  BreakpointsForDimension1Spacing=12  BreakpointsForDimension2Spacing=12  IndexSearchMethod=Linear search  BeginIndexSearchUsingPreviousIndexResult=on  Table=db.aerody.CLDEM  ExtrapMethod=Clip  DiagnosticForOutOfRangeInput=Warning  InternalRulePriority=Speed  RndMeth=Simplest
      settings: InputPortMap=u0,u1
  Product : Product
  Sum : Sum  Inputs=19
  CL1 : Outport
  wires:
  BusElementIn7/1 -> 2-D Lookup Table16/3, 2-D Lookup Table1/1
  BusElementIn1/1 -> 2-D Lookup Table17/3, 2-D Lookup Table6/1
  BusElementIn2/1 -> 2-D Lookup Table18/3, 2-D Lookup Table2/1
  BusElementIn3/1 -> 2-D Lookup Table19/3, 2-D Lookup Table3/1
  BusElementIn4/1 -> 2-D Lookup Table4/1
  BusElementIn5/1 -> 2-D Lookup Table5/1
  BusElementIn6/1 -> 2-D Lookup Table8/1
  BusElementIn8/1 -> 2-D Lookup Table9/1
  BusElementIn9/1 -> 2-D Lookup Table10/1
  BusElementIn10/1 -> 2-D Lookup Table13/1, 2-D Lookup Table12/1
  beta/1 -> 2-D Lookup Table13/3, Product/2, 2-D Lookup Table/1
  2-D Lookup Table/1 -> Product/1
  height/1 -> 2-D Lookup Table19/1, 2-D Lookup Table18/1, 2-D Lookup Table17/1, 2-D Lookup Table16/1, 2-D Lookup Table15/1
  TC/1 -> 2-D Lookup Table20/1
  alpha/1 -> 2-D Lookup Table12/2, 2-D Lookup Table13/2, 2-D Lookup Table/2, 2-D Lookup Table10/2, 2-D Lookup Table9/2, 2-D Lookup Table8/2, 2-D Lookup Table5/2, 2-D Lookup Table4/2, 2-D Lookup Table3/2, 2-D Lookup Table2/2, 2-D Lookup Table6/2, 2-D Lookup Table1/2, 2-D Lookup Table19/2, 2-D Lookup Table18/2, 2-D Lookup Table17/2, 2-D Lookup Table16/2, 2-D Lookup Table15/2, 2-D Lookup Table20/2, 2-D Lookup Table7/1
  2-D Lookup Table2/1 -> Sum/10  "CLDFRI"
  2-D Lookup Table4/1 -> Sum/12  "CLDAL"
  2-D Lookup Table3/1 -> Sum/11  "CLDFRO"
  2-D Lookup Table1/1 -> Sum/8  "CLDFLI"
  2-D Lookup Table6/1 -> Sum/9  "CLDFLO"
  2-D Lookup Table8/1 -> Sum/14  "CLDEL"
  2-D Lookup Table18/1 -> Sum/6  "CLHDFRI"
  2-D Lookup Table5/1 -> Sum/13  "CLDAR"
  2-D Lookup Table19/1 -> Sum/7  "CLHDFRO"
  2-D Lookup Table10/1 -> Sum/16  "CLDER"
  2-D Lookup Table16/1 -> Sum/4  "CLHDFLI"
  2-D Lookup Table9/1 -> Sum/15  "CLDEM"
  2-D Lookup Table17/1 -> Sum/5  "CLHDFLO"
  2-D Lookup Table12/1 -> Sum/17  "CLDR"
  2-D Lookup Table20/1 -> Sum/2  "CLSS"
  Product/1 -> Sum/18  "DCLBETA*BETA"
  2-D Lookup Table15/1 -> Sum/3  "CLH"
  2-D Lookup Table7/1 -> Sum/1  "CLB"
  2-D Lookup Table13/1 -> Sum/19  "CLDRBETA"
  Sum/1 -> CL1/1
